simulink model "SWC_CDD_type"  (R2021b)
settings: Solver=FixedStepDiscrete  StartTime=0.0  StopTime=10.0  RelTol=1e-3
settings Model: DataDictionary=APPTypes.sldd  Creator=FVT23010  LastModifiedBy=FVT23010
settings DataIOCC: SaveFormat=StructureWithTime
settings OptimizationCC: DefaultParameterBehavior=Inlined  EnhancedBackFolding=on  PassReuseOutputArgsAs=Individual arguments  ZeroExternalMemoryAtStartup=off  ZeroInternalMemoryAtStartup=off  OptimizeBlockOrder=speed  DifferentSizesBufferReuse=on  OptimizationCustomize=off  EfficientTunableParamExpr=on
settings DebuggingCC: ParameterTunabilityLossMsg=error
settings HardwareCC: ProdBitPerPointer=32  ProdBitPerSizeT=32  ProdBitPerPtrDiffT=32  ProdLargestAtomicInteger=Long  ProdLargestAtomicFloat=Double  ProdWordSize=32  ProdLongLongMode=on  ProdHWDeviceType=ARM Compatible->ARM Cortex-M
settings SFSimCC: MATLABDynamicMemAlloc=off
settings RTWCC: Description=AUTOSAR  SystemTargetFile=autosar.tlc  GenCodeOnly=on  TemplateMakefile=ert_default_tmf  PortableWordSizes=on
settings CodeAppCC: ForceParamTrailComments=on  IgnoreCustomStorageClasses=off  OperatorAnnotations=on  SimulinkDataObjDesc=on  SFDataObjDesc=on  InsertBlockDesc=on
settings STFCustomTargetCC: TargetLangStandard=C99 (ISO)  MultiwordLength=256  ParMdlRefBuildCompliant=on  CompOptLevelCompliant=on  IncludeMdlTerminateFcn=off  CombineOutputUpdateFcns=on  SuppressErrorStatus=on  ERTCustomFileBanners=on  SupportNonFinite=off  SupportComplex=off  SupportContinuousTime=off  SupportNonInlinedSFcns=off  RemoveResetFunc=on  MATLABClassNameForMDSCustomization=Simulink.SoftwareTarget.ERTCustomization  AutosarCompliant=on  GRTInterface=off  UseToolchainInfoCompliant=on  LookupTableObjectStructAxisOrder=2,1,3,4,...  LUTObjectStructOrderEvenSpacing=Size,Table,Breakpoints  SystemTargetFile=autosar.tlc
settings ERTTargetCC: TargetLangStandard=C99 (ISO)  ConcurrentExecutionCompliant=off  IncludeMdlTerminateFcn=off  SuppressErrorStatus=on  SupportNonFinite=off  SupportComplex=off  ModelStepFunctionPrototypeControlCompliant=off  CPPClassGenCompliant=off  AutosarCompliant=on  LookupTableObjectStructAxisOrder=2,1,3,4,...  LUTObjectStructOrderEvenSpacing=Size,Table,Breakpoints  GenerateASAP2=on  InlinedParameterPlacement=NonHierarchical  ERTCustomFileTemplate=example_file_process.tlc  ConvertIfToSwitch=off  SuppressUnreachableDefaultCases=off  BooleanTrueId=true_MatlabRTW  BooleanFalseId=false_MatlabRTW

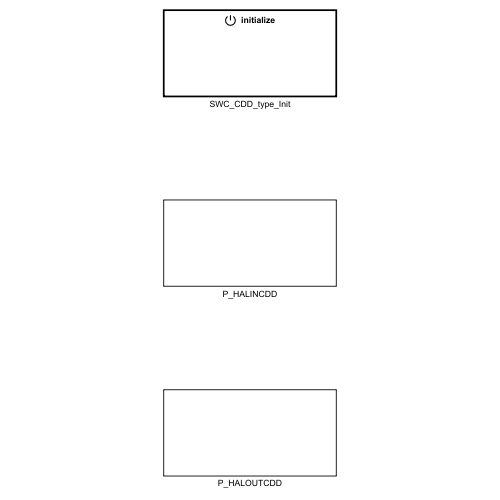
[thumbnail: Simulink's stored preview of the top-level diagram]
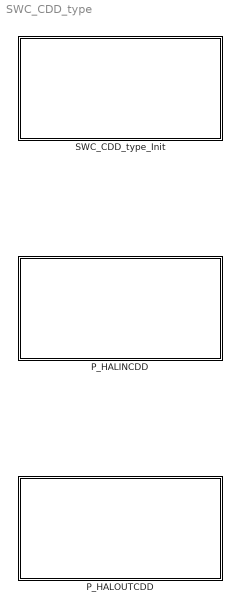
== system SWC_CDD_type ==
  P_HALINCDD : Subsystem
  P_HALOUTCDD : Subsystem
  SWC_CDD_type_Init : Subsystem

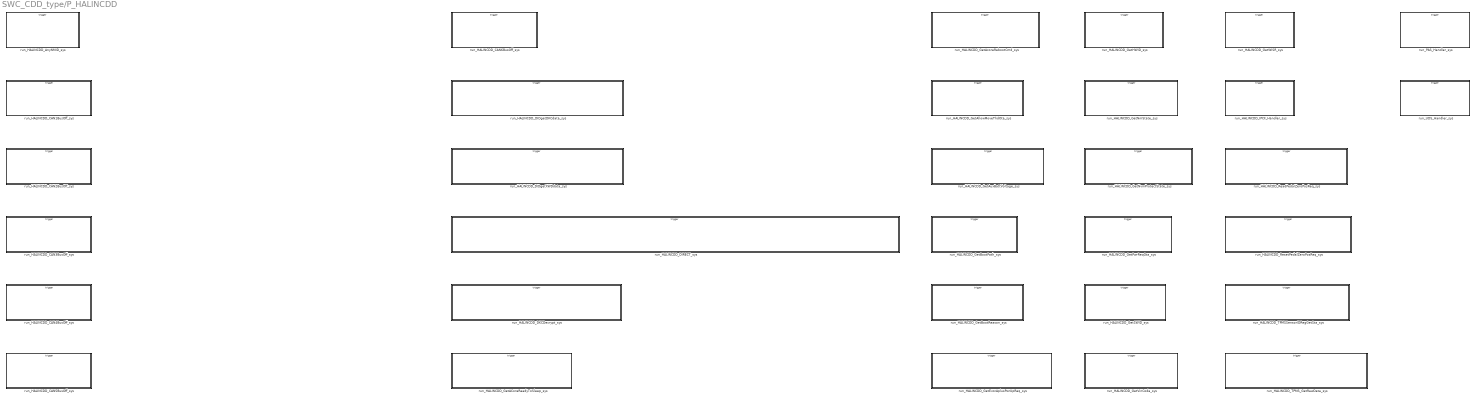
== system SWC_CDD_type/P_HALINCDD ==
  run_HALINCDD_AnyNMID_sys : Subsystem
  run_HALINCDD_CAN1BusOff_sys : Subsystem
  run_HALINCDD_CAN2BusOff_sys : Subsystem
  run_HALINCDD_CAN3BusOff_sys : Subsystem
  run_HALINCDD_CAN4BusOff_sys : Subsystem
  run_HALINCDD_CAN5BusOff_sys : Subsystem
  run_HALINCDD_CAN6BusOff_sys : Subsystem
  run_HALINCDD_DIDgetDKCdata_sys : Subsystem
  run_HALINCDD_DIDgetXWDdata_sys : Subsystem
  run_HALINCDD_DIRECT_sys : Subsystem
  run_HALINCDD_DKCDecrypt_sys : Subsystem
  run_HALINCDD_GetACoreReadyToSleep_sys : Subsystem
  run_HALINCDD_GetAcoreRebootCmd_sys : Subsystem
  run_HALINCDD_GetAllowMoveThdOta_sys : Subsystem
  run_HALINCDD_GetAuxBattVoltage_sys : Subsystem
  run_HALINCDD_GetBootPath_sys : Subsystem
  run_HALINCDD_GetBootReason_sys : Subsystem
  run_HALINCDD_GetEvccAplusPwrUpReq_sys : Subsystem
  run_HALINCDD_GetHWID_sys : Subsystem
  run_HALINCDD_GetNmState_sys : Subsystem
  run_HALINCDD_GetNvmProtectState_sys : Subsystem
  run_HALINCDD_GetPwrReqOta_sys : Subsystem
  run_HALINCDD_GetSWID_sys : Subsystem
  run_HALINCDD_GetVinCode_sys : Subsystem
  run_HALINCDD_GetWISR_sys : Subsystem
  run_HALINCDD_IPCF_Handler_sys : Subsystem
  run_HALINCDD_ReadPedalZeroPosReq_sys : Subsystem
  run_HALINCDD_ResetPedalZeroPosReq_sys : Subsystem
  run_HALINCDD_TPMSSensorIDRegGetSta_sys : Subsystem
  run_HALINCDD_TPMS_GetRawData_sys : Subsystem
  run_PAS_Handler_sys : Subsystem
  run_UDS_Handler_sys : Subsystem

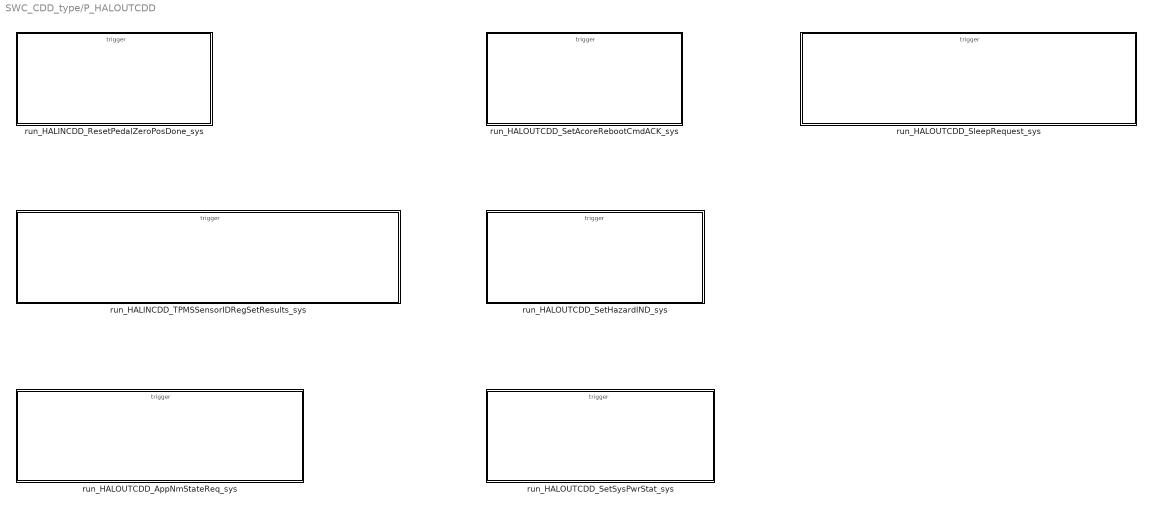
== system SWC_CDD_type/P_HALOUTCDD ==
  run_HALINCDD_ResetPedalZeroPosDone_sys : Subsystem
  run_HALINCDD_TPMSSensorIDRegSetResults_sys : Subsystem
  run_HALOUTCDD_AppNmStateReq_sys : Subsystem
  run_HALOUTCDD_SetAcoreRebootCmdACK_sys : Subsystem
  run_HALOUTCDD_SetHazardIND_sys : Subsystem
  run_HALOUTCDD_SetSysPwrStat_sys : Subsystem
  run_HALOUTCDD_SleepRequest_sys : Subsystem

== system SWC_CDD_type/SWC_CDD_type_Init ==
  Event Listener : EventListener  EventName=reset

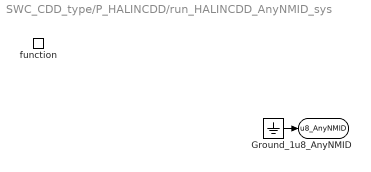
== system SWC_CDD_type/P_HALINCDD/run_HALINCDD_AnyNMID_sys ==
  function : TriggerPort  TriggerType=function-call  IsSimulinkFunction=on  FunctionName=run_HALINCDD_AnyNMID  VariantControl=(inherit)
  Ground_1 : Ground
  u8_AnyNMID : ArgOut  OutDataTypeStr=uint8  ArgumentName=u8_AnyNMID
  wires:
  Ground_1/1 -> u8_AnyNMID/1

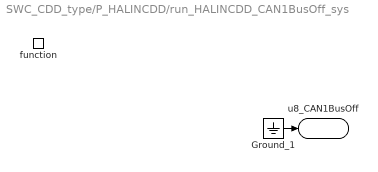
== system SWC_CDD_type/P_HALINCDD/run_HALINCDD_CAN1BusOff_sys ==
  function : TriggerPort  TriggerType=function-call  IsSimulinkFunction=on  FunctionName=run_HALINCDD_CAN1BusOff  VariantControl=(inherit)
  Ground_1 : Ground
  u8_CAN1BusOff : ArgOut  OutDataTypeStr=uint8  ArgumentName=u8_CAN1BusOff
  wires:
  Ground_1/1 -> u8_CAN1BusOff/1

== system SWC_CDD_type/P_HALINCDD/run_HALINCDD_CAN2BusOff_sys ==
  function : TriggerPort  TriggerType=function-call  IsSimulinkFunction=on  FunctionName=run_HALINCDD_CAN2BusOff  VariantControl=(inherit)
  Ground_1 : Ground
  u8_CAN2BusOff : ArgOut  OutDataTypeStr=uint8  ArgumentName=u8_CAN2BusOff
  wires:
  Ground_1/1 -> u8_CAN2BusOff/1

== system SWC_CDD_type/P_HALINCDD/run_HALINCDD_CAN3BusOff_sys ==
  function : TriggerPort  TriggerType=function-call  IsSimulinkFunction=on  FunctionName=run_HALINCDD_CAN3BusOff  VariantControl=(inherit)
  Ground_1 : Ground
  u8_CAN3BusOff : ArgOut  OutDataTypeStr=uint8  ArgumentName=u8_CAN3BusOff
  wires:
  Ground_1/1 -> u8_CAN3BusOff/1

== system SWC_CDD_type/P_HALINCDD/run_HALINCDD_CAN4BusOff_sys ==
  function : TriggerPort  TriggerType=function-call  IsSimulinkFunction=on  FunctionName=run_HALINCDD_CAN4BusOff  VariantControl=(inherit)
  Ground_1 : Ground
  u8_CAN4BusOff : ArgOut  OutDataTypeStr=uint8  ArgumentName=u8_CAN4BusOff
  wires:
  Ground_1/1 -> u8_CAN4BusOff/1

== system SWC_CDD_type/P_HALINCDD/run_HALINCDD_CAN5BusOff_sys ==
  function : TriggerPort  TriggerType=function-call  IsSimulinkFunction=on  FunctionName=run_HALINCDD_CAN5BusOff  VariantControl=(inherit)
  Ground_1 : Ground
  u8_CAN5BusOff : ArgOut  OutDataTypeStr=uint8  ArgumentName=u8_CAN5BusOff
  wires:
  Ground_1/1 -> u8_CAN5BusOff/1

== system SWC_CDD_type/P_HALINCDD/run_HALINCDD_CAN6BusOff_sys ==
  function : TriggerPort  TriggerType=function-call  IsSimulinkFunction=on  FunctionName=run_HALINCDD_CAN6BusOff  VariantControl=(inherit)
  Ground_1 : Ground
  u8_CAN6BusOff : ArgOut  OutDataTypeStr=uint8  ArgumentName=u8_CAN6BusOff
  wires:
  Ground_1/1 -> u8_CAN6BusOff/1

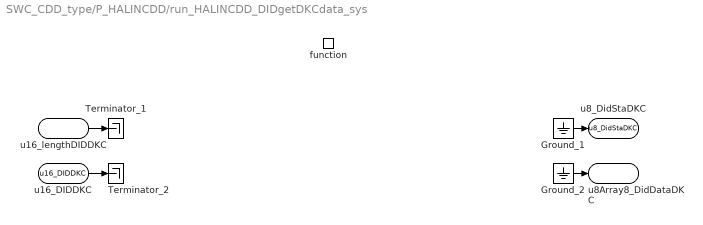
== system SWC_CDD_type/P_HALINCDD/run_HALINCDD_DIDgetDKCdata_sys ==
  function : TriggerPort  TriggerType=function-call  IsSimulinkFunction=on  FunctionName=run_DIDgetDKCdata  VariantControl=(inherit)
  Ground_1 : Ground
  Ground_2 : Ground
  Terminator_1 : Terminator
  Terminator_2 : Terminator
  u16_lengthDIDDKC : ArgIn  OutDataTypeStr=uint16  ArgumentName=u16_lengthDIDDKC
  u16_DIDDKC : ArgIn  Port=2  OutDataTypeStr=uint16  ArgumentName=u16_DIDDKC
  u8_DidStaDKC : ArgOut  OutDataTypeStr=uint8  ArgumentName=u8_DidStaDKC
  u8Array8_DidDataDKC : ArgOut  Port=2  OutDataTypeStr=uint8  PortDimensions=8  ArgumentName=u8Array8_DidDataDKC
  wires:
  u16_lengthDIDDKC/1 -> Terminator_1/1
  u16_DIDDKC/1 -> Terminator_2/1
  Ground_1/1 -> u8_DidStaDKC/1
  Ground_2/1 -> u8Array8_DidDataDKC/1

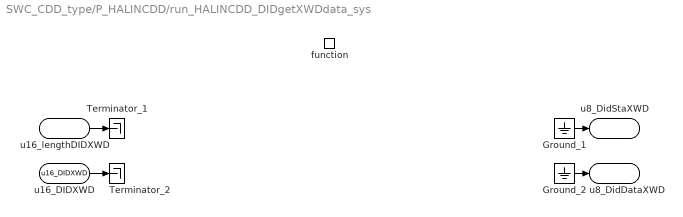
== system SWC_CDD_type/P_HALINCDD/run_HALINCDD_DIDgetXWDdata_sys ==
  function : TriggerPort  TriggerType=function-call  IsSimulinkFunction=on  FunctionName=run_HALINCDD_GetDIDdata  VariantControl=(inherit)
  Ground_1 : Ground
  Ground_2 : Ground
  Terminator_1 : Terminator
  Terminator_2 : Terminator
  u16_lengthDIDXWD : ArgIn  OutDataTypeStr=uint16  ArgumentName=u16_lengthDIDXWD
  u16_DIDXWD : ArgIn  Port=2  OutDataTypeStr=uint16  ArgumentName=u16_DIDXWD
  u8_DidStaXWD : ArgOut  OutDataTypeStr=uint8  ArgumentName=u8_DidStaXWD
  u8_DidDataXWD : ArgOut  Port=2  OutDataTypeStr=uint8  ArgumentName=u8_DidDataXWD
  wires:
  u16_lengthDIDXWD/1 -> Terminator_1/1
  u16_DIDXWD/1 -> Terminator_2/1
  Ground_1/1 -> u8_DidStaXWD/1
  Ground_2/1 -> u8_DidDataXWD/1

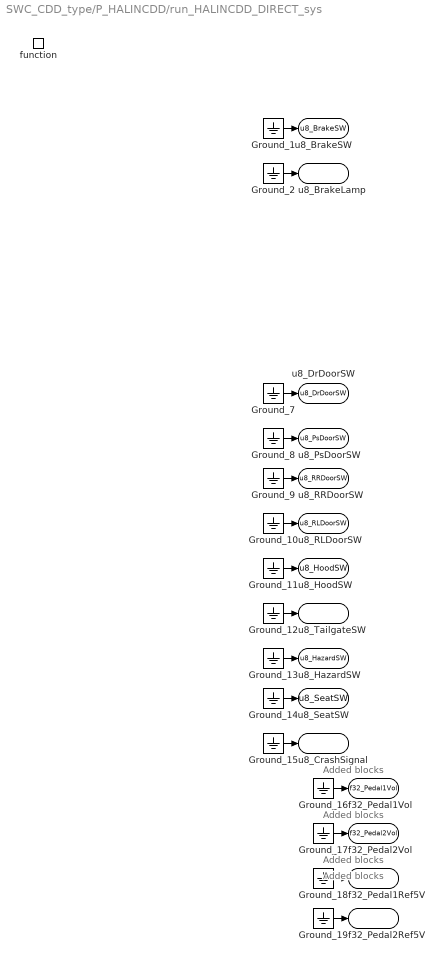
== system SWC_CDD_type/P_HALINCDD/run_HALINCDD_DIRECT_sys ==
  note: Added blocks
  note: Added blocks
  note: Added blocks
  note: Added blocks
  function : TriggerPort  TriggerType=function-call  IsSimulinkFunction=on  FunctionName=run_HALINCDD_DIRECT  VariantControl=(inherit)
  Ground_{1..2,7..19} (15 alike) : Ground
  u8_BrakeSW : ArgOut  OutDataTypeStr=uint8  ArgumentName=u8_BrakeSW
  u8_BrakeLamp : ArgOut  Port=2  OutDataTypeStr=uint8  ArgumentName=u8_BrakeLamp
  u8_DrDoorSW : ArgOut  Port=3  OutDataTypeStr=uint8  ArgumentName=u8_DrDoorSW
  u8_PsDoorSW : ArgOut  Port=4  OutDataTypeStr=uint8  ArgumentName=u8_PsDoorSW
  u8_RRDoorSW : ArgOut  Port=5  OutDataTypeStr=uint8  ArgumentName=u8_RRDoorSW
  u8_RLDoorSW : ArgOut  Port=6  OutDataTypeStr=uint8  ArgumentName=u8_RLDoorSW
  u8_HoodSW : ArgOut  Port=7  OutDataTypeStr=uint8  ArgumentName=u8_HoodSW
  u8_TailgateSW : ArgOut  Port=8  OutDataTypeStr=uint8  ArgumentName=u8_TailgateSW
  u8_HazardSW : ArgOut  Port=9  OutDataTypeStr=uint8  ArgumentName=u8_HazardSW
  u8_SeatSW : ArgOut  Port=10  OutDataTypeStr=uint8  ArgumentName=u8_SeatSW
  u8_CrashSignal : ArgOut  Port=11  OutDataTypeStr=uint8  ArgumentName=u8_CrashSignal
  f32_Pedal1Vol : ArgOut  Port=12  OutDataTypeStr=single  ArgumentName=f32_Pedal1Vol
  f32_Pedal2Vol : ArgOut  Port=13  OutDataTypeStr=single  ArgumentName=f32_Pedal2Vol
  f32_Pedal1Ref5V : ArgOut  Port=14  OutDataTypeStr=single  ArgumentName=f32_Pedal1Ref5V
  f32_Pedal2Ref5V : ArgOut  Port=15  OutDataTypeStr=single  ArgumentName=f32_Pedal2Ref5V
  wires:
  Ground_1/1 -> u8_BrakeSW/1
  Ground_2/1 -> u8_BrakeLamp/1
  Ground_7/1 -> u8_DrDoorSW/1
  Ground_8/1 -> u8_PsDoorSW/1
  Ground_9/1 -> u8_RRDoorSW/1
  Ground_10/1 -> u8_RLDoorSW/1
  Ground_11/1 -> u8_HoodSW/1
  Ground_12/1 -> u8_TailgateSW/1
  Ground_13/1 -> u8_HazardSW/1
  Ground_14/1 -> u8_SeatSW/1
  Ground_15/1 -> u8_CrashSignal/1
  Ground_16/1 -> f32_Pedal1Vol/1
  Ground_17/1 -> f32_Pedal2Vol/1
  Ground_18/1 -> f32_Pedal1Ref5V/1
  Ground_19/1 -> f32_Pedal2Ref5V/1

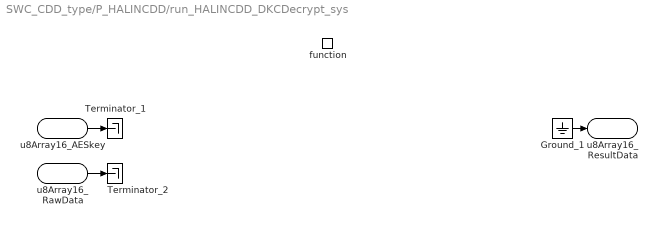
== system SWC_CDD_type/P_HALINCDD/run_HALINCDD_DKCDecrypt_sys ==
  function : TriggerPort  TriggerType=function-call  IsSimulinkFunction=on  FunctionName=run_HALINCDD_DKCDecrypt  VariantControl=(inherit)
  Ground_1 : Ground
  Terminator_1 : Terminator
  Terminator_2 : Terminator
  u8Array16_AESkey : ArgIn  OutDataTypeStr=uint8  PortDimensions=16  ArgumentName=u8Array16_AESkey
  u8Array16_RawData : ArgIn  Port=2  OutDataTypeStr=uint8  PortDimensions=16  ArgumentName=u8Array16_RawData
  u8Array16_ResultData : ArgOut  OutDataTypeStr=uint8  PortDimensions=16  ArgumentName=u8Array16_ResultData
  wires:
  u8Array16_AESkey/1 -> Terminator_1/1
  u8Array16_RawData/1 -> Terminator_2/1
  Ground_1/1 -> u8Array16_ResultData/1

== system SWC_CDD_type/P_HALINCDD/run_HALINCDD_GetACoreReadyToSleep_sys ==
  function : TriggerPort  TriggerType=function-call  IsSimulinkFunction=on  FunctionName=run_HALINCDD_GetACoreReadyToSleep  VariantControl=(inherit)
  Ground_1 : Ground
  s8_AcoreReadyToSleep : ArgOut  OutDataTypeStr=int8  ArgumentName=s8_AcoreReadyToSleep
  wires:
  Ground_1/1 -> s8_AcoreReadyToSleep/1

== system SWC_CDD_type/P_HALINCDD/run_HALINCDD_GetAcoreRebootCmd_sys ==
  function : TriggerPort  TriggerType=function-call  IsSimulinkFunction=on  FunctionName=run_HALINCDD_GetAcoreRebootCmd  VariantControl=(inherit)
  Ground_1 : Ground
  u8_AcoreRebootCmd : ArgOut  OutDataTypeStr=uint8  ArgumentName=u8_AcoreRebootCmd
  wires:
  Ground_1/1 -> u8_AcoreRebootCmd/1

== system SWC_CDD_type/P_HALINCDD/run_HALINCDD_GetAllowMoveThdOta_sys ==
  function : TriggerPort  TriggerType=function-call  IsSimulinkFunction=on  FunctionName=run_GetAllowMoveThdOta  VariantControl=(inherit)
  Ground_1 : Ground
  u8_AllowMovThdOTA : ArgOut  OutDataTypeStr=uint8  ArgumentName=u8_AllowMovThdOTA
  wires:
  Ground_1/1 -> u8_AllowMovThdOTA/1

== system SWC_CDD_type/P_HALINCDD/run_HALINCDD_GetAuxBattVoltage_sys ==
  function : TriggerPort  TriggerType=function-call  IsSimulinkFunction=on  FunctionName=run_HALINCDD_GetAuxBattVoltage  VariantControl=(inherit)
  Ground_1 : Ground
  u16_AuxBattVol100mV : ArgOut  OutDataTypeStr=uint16  ArgumentName=u16_AuxBattVol100mV
  wires:
  Ground_1/1 -> u16_AuxBattVol100mV/1

== system SWC_CDD_type/P_HALINCDD/run_HALINCDD_GetBootPath_sys ==
  function : TriggerPort  TriggerType=function-call  IsSimulinkFunction=on  FunctionName=run_HALINCDD_GetBootPath  VariantControl=(inherit)
  Ground_1 : Ground
  u32_BootPath : ArgOut  OutDataTypeStr=uint32  ArgumentName=u32_BootPath
  wires:
  Ground_1/1 -> u32_BootPath/1

== system SWC_CDD_type/P_HALINCDD/run_HALINCDD_GetBootReason_sys ==
  function : TriggerPort  TriggerType=function-call  IsSimulinkFunction=on  FunctionName=run_HALINCDD_GetBootReason  VariantControl=(inherit)
  Ground_1 : Ground
  u8_BootReason : ArgOut  OutDataTypeStr=uint8  ArgumentName=u8_BootReason
  wires:
  Ground_1/1 -> u8_BootReason/1

== system SWC_CDD_type/P_HALINCDD/run_HALINCDD_GetEvccAplusPwrUpReq_sys ==
  function : TriggerPort  TriggerType=function-call  IsSimulinkFunction=on  FunctionName=run_HALINCDD_GetEvccAplusPwrUpReq  VariantControl=(inherit)
  Ground_1 : Ground
  u8_EvccAplusPwrUpReq : ArgOut  OutDataTypeStr=uint8  ArgumentName=u8_EvccAplusPwrUpReq
  wires:
  Ground_1/1 -> u8_EvccAplusPwrUpReq/1

== system SWC_CDD_type/P_HALINCDD/run_HALINCDD_GetHWID_sys ==
  function : TriggerPort  TriggerType=function-call  IsSimulinkFunction=on  FunctionName=run_HALINCDD_GetHWID  VariantControl=(inherit)
  Ground_1 : Ground
  u8Array4_HWID : ArgOut  OutDataTypeStr=uint8  PortDimensions=4  ArgumentName=u8Array4_HWID
  wires:
  Ground_1/1 -> u8Array4_HWID/1

== system SWC_CDD_type/P_HALINCDD/run_HALINCDD_GetNmState_sys ==
  function : TriggerPort  TriggerType=function-call  IsSimulinkFunction=on  FunctionName=run_HALINCDD_GetNmState  VariantControl=(inherit)
  Ground_1 : Ground
  u8_CurrentNMState : ArgOut  OutDataTypeStr=uint8  ArgumentName=u8_CurrentNMState
  wires:
  Ground_1/1 -> u8_CurrentNMState/1

== system SWC_CDD_type/P_HALINCDD/run_HALINCDD_GetNvmProtectState_sys ==
  function : TriggerPort  TriggerType=function-call  IsSimulinkFunction=on  FunctionName=run_HALINCDD_GetNvmProtectState  VariantControl=(inherit)
  Ground_1 : Ground
  u8_NvmProtectSta : ArgOut  OutDataTypeStr=uint8  ArgumentName=u8_NvmProtectSta
  wires:
  Ground_1/1 -> u8_NvmProtectSta/1

== system SWC_CDD_type/P_HALINCDD/run_HALINCDD_GetPwrReqOta_sys ==
  function : TriggerPort  TriggerType=function-call  IsSimulinkFunction=on  FunctionName=run_HALINCDD_GetPwrReqOta  VariantControl=(inherit)
  Ground_1 : Ground
  u8_PwrReqOTA : ArgOut  OutDataTypeStr=uint8  ArgumentName=u8_PwrReqOTA
  wires:
  Ground_1/1 -> u8_PwrReqOTA/1

== system SWC_CDD_type/P_HALINCDD/run_HALINCDD_GetSWID_sys ==
  function : TriggerPort  TriggerType=function-call  IsSimulinkFunction=on  FunctionName=run_HALINCDD_GetSWID  VariantControl=(inherit)
  Ground_1 : Ground
  u8Array33_SWID : ArgOut  OutDataTypeStr=uint8  PortDimensions=33  ArgumentName=u8Array33_SWID
  wires:
  Ground_1/1 -> u8Array33_SWID/1

== system SWC_CDD_type/P_HALINCDD/run_HALINCDD_GetVinCode_sys ==
  function : TriggerPort  TriggerType=function-call  IsSimulinkFunction=on  FunctionName=run_HALINCDD_GetVinCode  VariantControl=(inherit)
  Ground_1 : Ground
  u8Array17_VinCode : ArgOut  OutDataTypeStr=uint8  PortDimensions=17  ArgumentName=u8Array17_VinCode
  wires:
  Ground_1/1 -> u8Array17_VinCode/1

== system SWC_CDD_type/P_HALINCDD/run_HALINCDD_GetWISR_sys ==
  function : TriggerPort  TriggerType=function-call  IsSimulinkFunction=on  FunctionName=run_HALINCDD_GetWISR  VariantControl=(inherit)
  Ground_1 : Ground
  u32_WISR : ArgOut  OutDataTypeStr=uint32  ArgumentName=u32_WISR
  wires:
  Ground_1/1 -> u32_WISR/1

== system SWC_CDD_type/P_HALINCDD/run_HALINCDD_IPCF_Handler_sys ==
  function : TriggerPort  TriggerType=function-call  IsSimulinkFunction=on  FunctionName=run_HALINCDD_IPCF_Handler  VariantControl=(inherit)

== system SWC_CDD_type/P_HALINCDD/run_HALINCDD_ReadPedalZeroPosReq_sys ==
  function : TriggerPort  TriggerType=function-call  IsSimulinkFunction=on  FunctionName=run_HALINCDD_ReadPedalZeroPosReq  VariantControl=(inherit)
  Ground_1 : Ground
  u8_ReadPedalZeroPosReq : ArgOut  OutDataTypeStr=uint8  ArgumentName=u8_ReadPedalZeroPosReq
  wires:
  Ground_1/1 -> u8_ReadPedalZeroPosReq/1

== system SWC_CDD_type/P_HALINCDD/run_HALINCDD_ResetPedalZeroPosReq_sys ==
  function : TriggerPort  TriggerType=function-call  IsSimulinkFunction=on  FunctionName=run_HALINCDD_ResetPedalZeroPosReq  VariantControl=(inherit)
  Ground_1 : Ground
  u8_ResetPedalZeroPosReq : ArgOut  OutDataTypeStr=uint8  ArgumentName=u8_ResetPedalZeroPosReq
  wires:
  Ground_1/1 -> u8_ResetPedalZeroPosReq/1

== system SWC_CDD_type/P_HALINCDD/run_HALINCDD_TPMSSensorIDRegGetSta_sys ==
  function : TriggerPort  TriggerType=function-call  IsSimulinkFunction=on  FunctionName=run_HALINCDD_TPMSSensorIDRegGetSta  VariantControl=(inherit)
  Ground_1 : Ground
  u8_TPMSSensorIDRegSta : ArgOut  OutDataTypeStr=uint8  ArgumentName=u8_TPMSSensorIDRegSta
  wires:
  Ground_1/1 -> u8_TPMSSensorIDRegSta/1

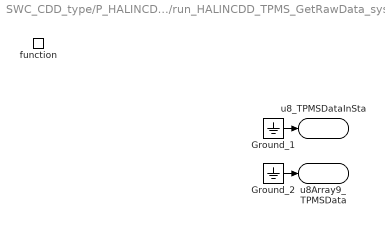
== system SWC_CDD_type/P_HALINCDD/run_HALINCDD_TPMS_GetRawData_sys ==
  function : TriggerPort  TriggerType=function-call  IsSimulinkFunction=on  FunctionName=run_HALINCDD_TPMS_GetRawData  VariantControl=(inherit)
  Ground_1 : Ground
  Ground_2 : Ground
  u8_TPMSDataInSta : ArgOut  OutDataTypeStr=boolean  ArgumentName=u8_TPMSDataInSta
  u8Array9_TPMSData : ArgOut  Port=2  OutDataTypeStr=uint8  PortDimensions=9  ArgumentName=u8Array9_TPMSData
  wires:
  Ground_1/1 -> u8_TPMSDataInSta/1
  Ground_2/1 -> u8Array9_TPMSData/1

== system SWC_CDD_type/P_HALINCDD/run_PAS_Handler_sys ==
  function : TriggerPort  TriggerType=function-call  IsSimulinkFunction=on  FunctionName=run_PAS_Handler  VariantControl=(inherit)

== system SWC_CDD_type/P_HALINCDD/run_UDS_Handler_sys ==
  function : TriggerPort  TriggerType=function-call  IsSimulinkFunction=on  FunctionName=run_UDS_Handler  VariantControl=(inherit)

== system SWC_CDD_type/P_HALOUTCDD/run_HALINCDD_ResetPedalZeroPosDone_sys ==
  function : TriggerPort  TriggerType=function-call  IsSimulinkFunction=on  FunctionName=run_HALINCDD_ResetPedalZeroPosDone  VariantControl=(inherit)

== system SWC_CDD_type/P_HALOUTCDD/run_HALINCDD_TPMSSensorIDRegSetResults_sys ==
  function : TriggerPort  TriggerType=function-call  IsSimulinkFunction=on  FunctionName=run_HALINCDD_TPMSSensorIDRegSetResults  VariantControl=(inherit)
  Terminator_1 : Terminator
  u8Array2_TPMSSensorIDRegResults : ArgIn  OutDataTypeStr=uint8  PortDimensions=2  ArgumentName=u8Array2_TPMSSensorIDRegResults
  wires:
  u8Array2_TPMSSensorIDRegResults/1 -> Terminator_1/1

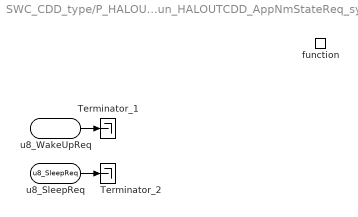
== system SWC_CDD_type/P_HALOUTCDD/run_HALOUTCDD_AppNmStateReq_sys ==
  function : TriggerPort  TriggerType=function-call  IsSimulinkFunction=on  FunctionName=run_HALOUTCDD_AppNmStateReq  VariantControl=(inherit)
  Terminator_1 : Terminator
  Terminator_2 : Terminator
  u8_WakeUpReq : ArgIn  OutDataTypeStr=uint8  ArgumentName=u8_WakeUpReq
  u8_SleepReq : ArgIn  Port=2  OutDataTypeStr=uint8  ArgumentName=u8_SleepReq
  wires:
  u8_WakeUpReq/1 -> Terminator_1/1
  u8_SleepReq/1 -> Terminator_2/1

== system SWC_CDD_type/P_HALOUTCDD/run_HALOUTCDD_SetAcoreRebootCmdACK_sys ==
  function : TriggerPort  TriggerType=function-call  IsSimulinkFunction=on  FunctionName=run_HALOUTCDD_SetAcoreRebootCmdACK  VariantControl=(inherit)

== system SWC_CDD_type/P_HALOUTCDD/run_HALOUTCDD_SetHazardIND_sys ==
  function : TriggerPort  TriggerType=function-call  IsSimulinkFunction=on  FunctionName=run_HALOUTCDD_SetHazardIND  VariantControl=(inherit)
  Terminator_1 : Terminator
  u8_HazardIND : ArgIn  OutDataTypeStr=uint8  ArgumentName=u8_HazardIND
  wires:
  u8_HazardIND/1 -> Terminator_1/1

== system SWC_CDD_type/P_HALOUTCDD/run_HALOUTCDD_SetSysPwrStat_sys ==
  function : TriggerPort  TriggerType=function-call  IsSimulinkFunction=on  FunctionName=run_HALOUTCDD_SetSysPwrStat  VariantControl=(inherit)
  Terminator_1 : Terminator
  u8_SysPwrStat : ArgIn  OutDataTypeStr=uint8  ArgumentName=u8_SysPwrStat
  wires:
  u8_SysPwrStat/1 -> Terminator_1/1

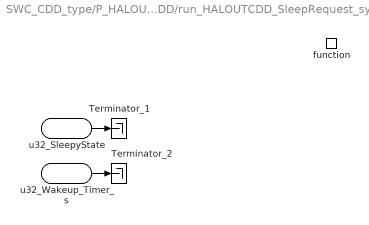
== system SWC_CDD_type/P_HALOUTCDD/run_HALOUTCDD_SleepRequest_sys ==
  function : TriggerPort  TriggerType=function-call  IsSimulinkFunction=on  FunctionName=run_HALOUTCDD_SleepRequest  VariantControl=(inherit)
  Terminator_1 : Terminator
  Terminator_2 : Terminator
  u32_SleepyState : ArgIn  OutDataTypeStr=uint32  ArgumentName=u32_SleepyState
  u32_Wakeup_Timer_s : ArgIn  Port=2  OutDataTypeStr=uint32  ArgumentName=u32_Wakeup_Timer_s
  wires:
  u32_SleepyState/1 -> Terminator_1/1
  u32_Wakeup_Timer_s/1 -> Terminator_2/1
